simulink model "s_freib"  (Simulink 4.00)
settings: Solver=ode45  SolverMode=SingleTasking  StartTime=0.0  StopTime=2  MaxStep=0.001  RelTol=1e-3  AbsTol=1e-6
settings Model: LastModifiedBy=Administrator  SaveTime=off  SaveOutput=off  LimitDataPoints=off  BlockReductionOpt=off

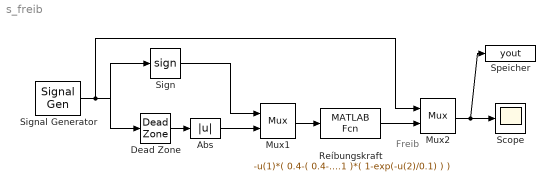
== system s_freib ==
  note: Freib
  Abs : Abs  SaturateOnIntegerOverflow=on
  Dead Zone : DeadZone  LowerValue=-0.1  UpperValue=0.1  SaturateOnIntegerOverflow=on  LinearizeAsGain=on
  Mux1 : Mux  Inputs=2
      settings: DisplayOption=none
  Mux2 : Mux  Inputs=2
      settings: DisplayOption=none
  Reíbungskraft : MATLABFcn  MATLABFcn=-u(1)*( 0.4-( 0.4-0.1 )*( 1-exp(-u(2)/0.1) ) )  OutputDimensions=1  OutputSignalType=auto  Output1D=on
  Scope : Scope
      settings: TickLabels=on  TimeRange=2.000000  YMin=-1.478  YMax=1.478  SaveToWorkspace=off  SaveName=ScopeData  DataFormat=Array  LimitDataPoints=on  MaxDataPoints=5000
  Sign : Signum
  Signal Generator : SignalGenerator  WaveForm=sawtooth  Amplitude=1.000000  Frequency=10.000000  Units=rad/sec
  Speicher : ToWorkspace  VariableName=yout  SampleTime=0  SaveFormat=Array
      settings: MaxDataPoints=1000
  wires:
  Mux2/1 -> Speicher/1, Scope/1
  Reíbungskraft/1 -> Mux2/2
  Signal Generator/1 -> Mux2/1, Dead Zone/1, Sign/1
  Dead Zone/1 -> Abs/1
  Abs/1 -> Mux1/2
  Mux1/1 -> Reíbungskraft/1
  Sign/1 -> Mux1/1
